simulink model "CalculatorSubSys"  (R2016a)
settings: Solver=FixedStepDiscrete  StartTime=0.0  StopTime=10.0  RelTol=1e-3
libraries: simulink x5
settings Model: Creator=Mohamed Fawzy  LastModifiedBy=Mohamed Fawzy
settings OptimizationCC: DefaultParameterBehavior=Inlined  OptimizeModelRefInitCode=on  LifeSpan=1
settings RTWCC: SystemTargetFile=ert.tlc  GenCodeOnly=on  GenerateMakefile=off  TemplateMakefile=ert_default_tmf  GenerateReport=on  IncludeHyperlinkInReport=on  LaunchReport=on  GenerateTraceInfo=on  GenerateTraceReport=on  GenerateTraceReportSl=on  GenerateTraceReportSf=on  GenerateTraceReportEml=on
settings CodeAppCC: ForceParamTrailComments=on  IgnoreCustomStorageClasses=off  OperatorAnnotations=on  SimulinkDataObjDesc=on  SFDataObjDesc=on  MATLABFcnDesc=on  InsertBlockDesc=on  MATLABSourceComments=on
settings ERTTargetCC: GenerateSampleERTMain=on  SuppressErrorStatus=on  InlinedParameterPlacement=NonHierarchical  ERTCustomFileTemplate=example_file_process.tlc

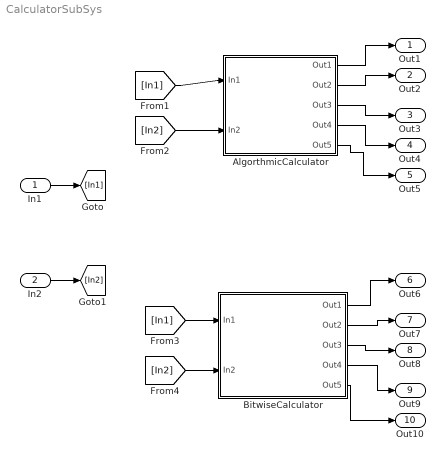
== system CalculatorSubSys ==
  In1 : Inport  OutDataTypeStr=uint8
  In2 : Inport  Port=2  OutDataTypeStr=uint8
  AlgorthmicCalculator : Subsystem  TreatAsAtomicUnit=on
      settings: RTWFcnNameOpts=Use subsystem name  RTWFileNameOpts=Use subsystem name
  BitwiseCalculator : Subsystem  TreatAsAtomicUnit=on
      settings: RTWFcnNameOpts=Use subsystem name  RTWFileNameOpts=Use subsystem name
  Out1 : Outport  OutDataTypeStr=uint8
  Out2 : Outport  Port=2  OutDataTypeStr=uint8
  Out3 : Outport  Port=3  OutDataTypeStr=uint16
  Out4 : Outport  Port=4  OutDataTypeStr=uint16
  Out5 : Outport  Port=5  OutDataTypeStr=uint8
  Out6 : Outport  Port=6  OutDataTypeStr=uint8
  Out7 : Outport  Port=7  OutDataTypeStr=uint8
  Out8 : Outport  Port=8  OutDataTypeStr=uint8
  Out9 : Outport  Port=9  OutDataTypeStr=uint8
  Out10 : Outport  Port=10  OutDataTypeStr=uint8
  wires:
  AlgorthmicCalculator/1(Out1) -> Out1/1
  AlgorthmicCalculator/2(Out2) -> Out2/1
  AlgorthmicCalculator/3(Out3) -> Out3/1
  AlgorthmicCalculator/4(Out4) -> Out4/1
  AlgorthmicCalculator/5(Out5) -> Out5/1
  [In1] -> AlgorthmicCalculator/1(In1)
  [In2] -> AlgorthmicCalculator/2(In2)
  BitwiseCalculator/1(Out1) -> Out6/1
  BitwiseCalculator/2(Out2) -> Out7/1
  BitwiseCalculator/3(Out3) -> Out8/1
  BitwiseCalculator/4(Out4) -> Out9/1
  BitwiseCalculator/5(Out5) -> Out10/1
  [In1] -> BitwiseCalculator/1(In1)
  [In2] -> BitwiseCalculator/2(In2)
  In1/1 -> [In1]
  In2/1 -> [In2]

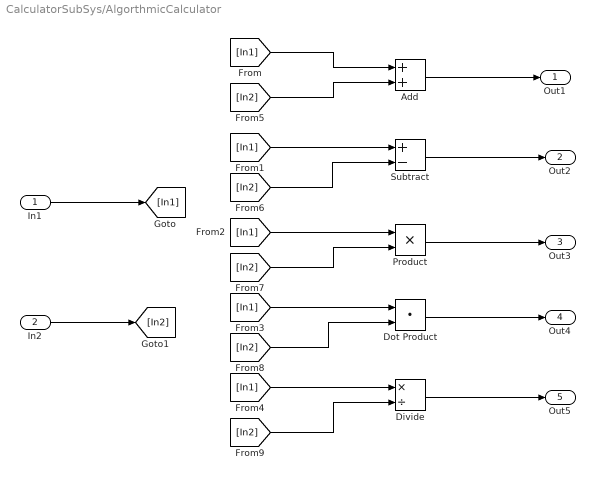
== system CalculatorSubSys/AlgorthmicCalculator ==
  In1 : Inport
  In2 : Inport  Port=2
  Add : Sum
  Divide : Product  Inputs=*/
  Dot Product : DotProduct  InputSameDT=on  OutDataTypeStr=Inherit: Inherit via internal rule
  Product : Product
  Subtract : Sum  Inputs=+-
  Out1 : Outport
  Out2 : Outport  Port=2
  Out3 : Outport  Port=3
  Out4 : Outport  Port=4
  Out5 : Outport  Port=5
  wires:
  [In2] -> Subtract/2
  Dot Product/1 -> Out4/1
  Add/1 -> Out1/1
  [In1] -> Product/1
  [In1] -> Add/1
  Subtract/1 -> Out2/1
  Divide/1 -> Out5/1
  [In1] -> Subtract/1
  Product/1 -> Out3/1
  [In1] -> Dot Product/1
  [In1] -> Divide/1
  [In2] -> Add/2
  In1/1 -> [In1]
  In2/1 -> [In2]
  [In2] -> Product/2
  [In2] -> Dot Product/2
  [In2] -> Divide/2

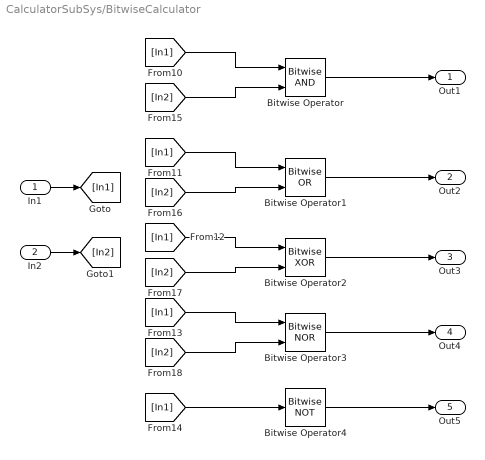
== system CalculatorSubSys/BitwiseCalculator ==
  In1 : Inport  OutDataTypeStr=uint8
  In2 : Inport  Port=2  OutDataTypeStr=uint8
  Bitwise Operator : simulink/Logic and Bit Operations/Bitwise Operator  logicop=AND  UseBitMask=off  NumInputPorts=2  BitMask=bin2dec('11011001')  BitMaskRealWorld=Stored Integer
  Bitwise Operator1 : simulink/Logic and Bit Operations/Bitwise Operator  logicop=OR  UseBitMask=off  NumInputPorts=2  BitMask=bin2dec('11011001')  BitMaskRealWorld=Stored Integer
  Bitwise Operator2 : simulink/Logic and Bit Operations/Bitwise Operator  logicop=XOR  UseBitMask=off  NumInputPorts=2  BitMask=bin2dec('11011001')  BitMaskRealWorld=Stored Integer
  Bitwise Operator3 : simulink/Logic and Bit Operations/Bitwise Operator  logicop=NOR  UseBitMask=off  NumInputPorts=2  BitMask=bin2dec('11011001')  BitMaskRealWorld=Stored Integer
  Bitwise Operator4 : simulink/Logic and Bit Operations/Bitwise Operator  logicop=NOT  UseBitMask=off  BitMask=bin2dec('11011001')  BitMaskRealWorld=Stored Integer
  Out1 : Outport
  Out2 : Outport  Port=2
  Out3 : Outport  Port=3
  Out4 : Outport  Port=4
  Out5 : Outport  Port=5
  wires:
  [In2] -> Bitwise Operator/2
  Bitwise Operator1/1 -> Out2/1
  Bitwise Operator2/1 -> Out3/1
  [In1] -> Bitwise Operator1/1
  [In2] -> Bitwise Operator3/2
  [In2] -> Bitwise Operator2/2
  Bitwise Operator/1 -> Out1/1
  Bitwise Operator3/1 -> Out4/1
  [In2] -> Bitwise Operator1/2
  Bitwise Operator4/1 -> Out5/1
  [In1] -> Bitwise Operator2/1
  In2/1 -> [In2]
  [In1] -> Bitwise Operator/1
  [In1] -> Bitwise Operator3/1
  [In1] -> Bitwise Operator4/1
  In1/1 -> [In1]
